simulink model "Kalman_Filter"  (R2025a)
settings: Solver=VariableStepAuto  StartTime=0.0  StopTime=10.0  RelTol=1e-3
settings Model: Creator=xing2  LastModifiedBy=xing2

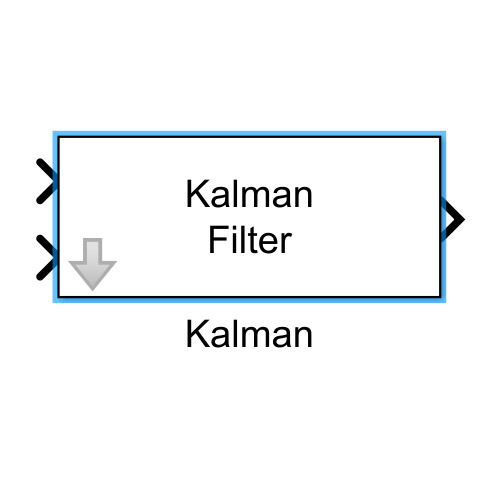
[thumbnail: Simulink's stored preview of the top-level diagram]
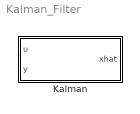
== system Kalman_Filter ==
  Kalman : Subsystem  mask{A_kf=[0 1;-10 -0.5], B_aug=[0 3;1 5], C_kf=[1 0;0 1], D_aug=[0 0;0 0], x0=[0;0]}
      mask prompts: A_kf "A matrix"; B_aug "B_aug=[B K]"; C_kf "C matrix"; D_aug "D matrix"
      mask help: Kalman Filter. B_aug=[B, K_kalman] for input [u; y]
      mask Display: disp('Kalman\nFilter');

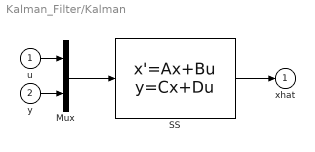
== system Kalman_Filter/Kalman ==
  u : Inport
  y : Inport  Port=2
  Mux : Mux  Inputs=2
  SS : StateSpace  A=A_kf  B=B_aug  C=C_kf  D=D_aug  InitialCondition=x0
  xhat : Outport
  wires:
  y/1 -> Mux/2
  u/1 -> Mux/1
  Mux/1 -> SS/1
  SS/1 -> xhat/1
